simulink model "projectCE1_v2"  (R2024a)
settings: Solver=VariableStepAuto  StartTime=0.0  StopTime=0.1  RelTol=1e-3
libraries: dspsrcs4 x9, dspfdesign x6, commanapbnd3 x3, commchan3 x1
settings Model: Creator=nagel  LastModifiedBy=nagel

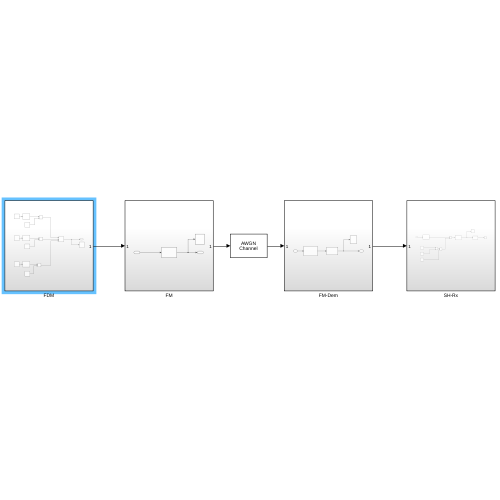
[thumbnail: Simulink's stored preview of the top-level diagram]
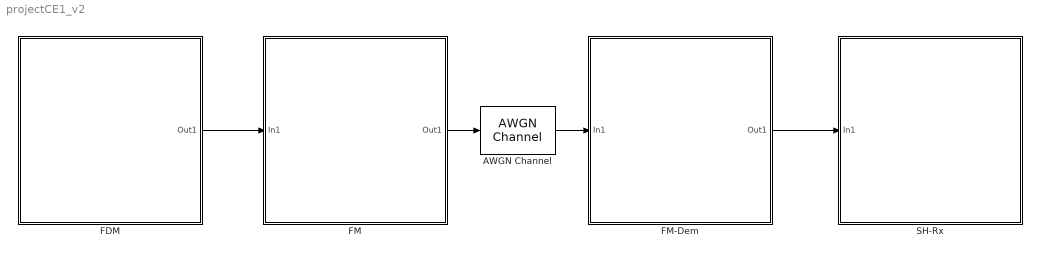
== system projectCE1_v2 ==
  AWGN Channel : commchan3/AWGN Channel  LegacyMode=off  NoiseMethod="Signal to noise ratio  (SNR)"  noiseMode="Signal to noise ratio  (SNR)"  EbNo=10  EsNo=10  SNR=10  BitsPerSymbol=1  SignalPower=1  SamplesPerSymbol=1  SymbolPeriod=1  VarianceSource=Parameter  Variance=1  RandomStream=mt19937ar with seed  Seed=67  SimulateUsing=Code generation
  FDM : Subsystem
  FM : Subsystem
  FM-Dem : Subsystem
  SH-Rx : Subsystem
  wires:
  FDM/1(Out1) -> FM/1(In1)
  FM/1(Out1) -> AWGN Channel/1
  AWGN Channel/1 -> FM-Dem/1(In1)
  FM-Dem/1(Out1) -> SH-Rx/1(In1)

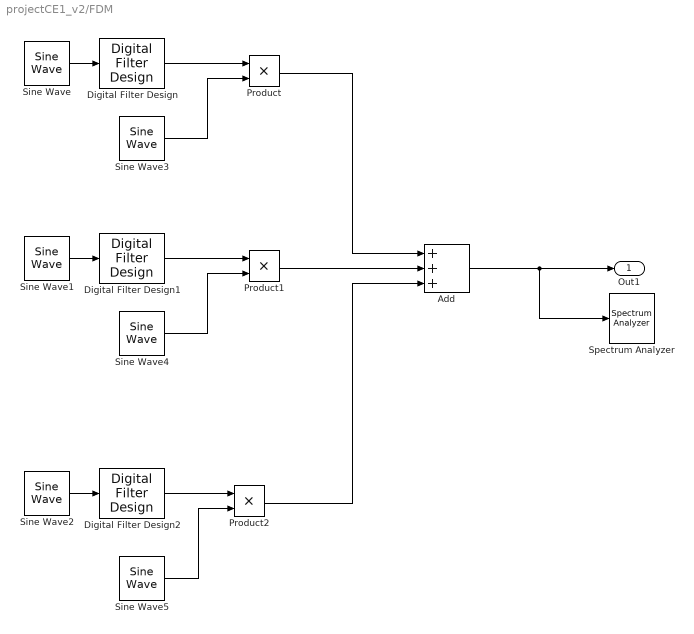
== system projectCE1_v2/FDM ==
  Add : Sum  Inputs=+++
  Digital Filter Design : dspfdesign/Digital Filter Design  mwdsp_browser_bugfix_var=off
  Digital Filter Design1 : dspfdesign/Digital Filter Design  mwdsp_browser_bugfix_var=off
  Digital Filter Design2 : dspfdesign/Digital Filter Design  mwdsp_browser_bugfix_var=off
  Product : Product
  Product1 : Product
  Product2 : Product
  Sine Wave : dspsrcs4/Sine Wave  Amplitude=1  Frequency=780  Phase=0  SampleMode=Discrete  OutComplex=Real  CompMethod=Trigonometric fcn  TableSize=Speed  SampleTime=1/(2*114e6)  SamplesPerFrame=1  ResetState=Restart at time zero  OutputFrames=off  dataType=double  wordLen=16  udDataType=sfix(16)  fracBitsMode=Best precision  numFracBits=15  OutDataTypeStr=double  LastOutDataTypeStr=double
  Sine Wave1 : dspsrcs4/Sine Wave  Amplitude=1  Frequency=4500  Phase=0  SampleMode=Discrete  OutComplex=Real  CompMethod=Trigonometric fcn  TableSize=Speed  SampleTime=1/(2*114e6)  SamplesPerFrame=1  ResetState=Restart at time zero  OutputFrames=off  dataType=double  wordLen=16  udDataType=sfix(16)  fracBitsMode=Best precision  numFracBits=15  OutDataTypeStr=double  LastOutDataTypeStr=double
  Sine Wave2 : dspsrcs4/Sine Wave  Amplitude=1  Frequency=10e3  Phase=0  SampleMode=Discrete  OutComplex=Real  CompMethod=Trigonometric fcn  TableSize=Speed  SampleTime=1/(2*114e6)  SamplesPerFrame=1  ResetState=Restart at time zero  OutputFrames=off  dataType=double  wordLen=16  udDataType=sfix(16)  fracBitsMode=Best precision  numFracBits=15  OutDataTypeStr=double  LastOutDataTypeStr=double
  Sine Wave3 : dspsrcs4/Sine Wave  Amplitude=1  Frequency=20e3  Phase=0  SampleMode=Discrete  OutComplex=Real  CompMethod=Trigonometric fcn  TableSize=Speed  SampleTime=1/(2*114e6)  SamplesPerFrame=1  ResetState=Restart at time zero  OutputFrames=off  dataType=double  wordLen=16  udDataType=sfix(16)  fracBitsMode=Best precision  numFracBits=15  OutDataTypeStr=double  LastOutDataTypeStr=double
  Sine Wave4 : dspsrcs4/Sine Wave  Amplitude=1  Frequency=60e3  Phase=0  SampleMode=Discrete  OutComplex=Real  CompMethod=Trigonometric fcn  TableSize=Speed  SampleTime=1/(2*114e6)  SamplesPerFrame=1  ResetState=Restart at time zero  OutputFrames=off  dataType=double  wordLen=16  udDataType=sfix(16)  fracBitsMode=Best precision  numFracBits=15  OutDataTypeStr=double  LastOutDataTypeStr=double
  Sine Wave5 : dspsrcs4/Sine Wave  Amplitude=1  Frequency=100e3  Phase=0  SampleMode=Discrete  OutComplex=Real  CompMethod=Trigonometric fcn  TableSize=Speed  SampleTime=1/(2*114e6)  SamplesPerFrame=1  ResetState=Restart at time zero  OutputFrames=off  dataType=double  wordLen=16  udDataType=sfix(16)  fracBitsMode=Best precision  numFracBits=15  OutDataTypeStr=double  LastOutDataTypeStr=double
  Spectrum Analyzer : SpectrumAnalyzer  WindowPosition=[372.000000,110.000000,1132.000000,588.000000,]  ScopeFrameLocation=window  SampleRate=44.1e3  PlotAsTwoSidedSpectrum=off  FrequencyScale=Log  FrequencySpan=Start and stop frequencies  Span=250e3  CenterFrequency=125e3  StartFrequency=0  StopFrequency=250e3  YLimits=[-44.5224692,27.38603855]
  Out1 : Outport
  wires:
  Sine Wave1/1 -> Digital Filter Design1/1
  Add/1 -> Out1/1, Spectrum Analyzer/1
  Sine Wave2/1 -> Digital Filter Design2/1
  Sine Wave/1 -> Digital Filter Design/1
  Digital Filter Design/1 -> Product/1
  Sine Wave3/1 -> Product/2
  Product/1 -> Add/1
  Digital Filter Design1/1 -> Product1/1
  Sine Wave4/1 -> Product1/2
  Product1/1 -> Add/2
  Sine Wave5/1 -> Product2/2
  Digital Filter Design2/1 -> Product2/1
  Product2/1 -> Add/3

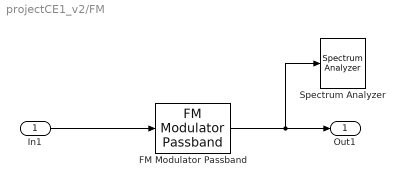
== system projectCE1_v2/FM ==
  In1 : Inport
  FM Modulator Passband : commanapbnd3/FM Modulator Passband  Fc=110e6  Ph=0  Kc=72e3
  Spectrum Analyzer : SpectrumAnalyzer  WindowPosition=[160.000000,154.000000,800.000000,500.000000,]  ScopeFrameLocation=window  RBWSource=Property  RBW=1e3  Span=227999999.99999997  StartFrequency=-113999999.99999999  StopFrequency=113999999.99999999  YLimits=[-99.98487156,25.09852185]
  Out1 : Outport
  wires:
  FM Modulator Passband/1 -> Spectrum Analyzer/1, Out1/1
  In1/1 -> FM Modulator Passband/1

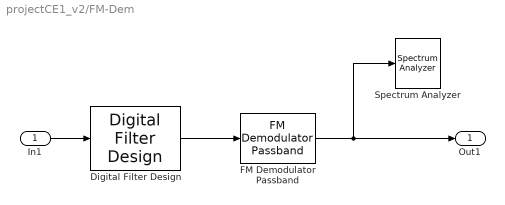
== system projectCE1_v2/FM-Dem ==
  In1 : Inport
  Digital Filter Design : dspfdesign/Digital Filter Design  mwdsp_browser_bugfix_var=off
  FM Demodulator Passband : commanapbnd3/FM Demodulator Passband  Fc=110e6  Ph=0  Kc=72e3  Ho=100
  Spectrum Analyzer : SpectrumAnalyzer  WindowPosition=[1027.000000,111.000000,800.000000,500.000000,]  ScopeFrameLocation=window  RBWSource=Property  RBW=1e3  Span=227999999.99999997  StartFrequency=-113999999.99999999  StopFrequency=113999999.99999999  YLimits=[-75.2783199,28.10619053]
  Out1 : Outport
  wires:
  In1/1 -> Digital Filter Design/1
  Digital Filter Design/1 -> FM Demodulator Passband/1
  FM Demodulator Passband/1 -> Spectrum Analyzer/1, Out1/1

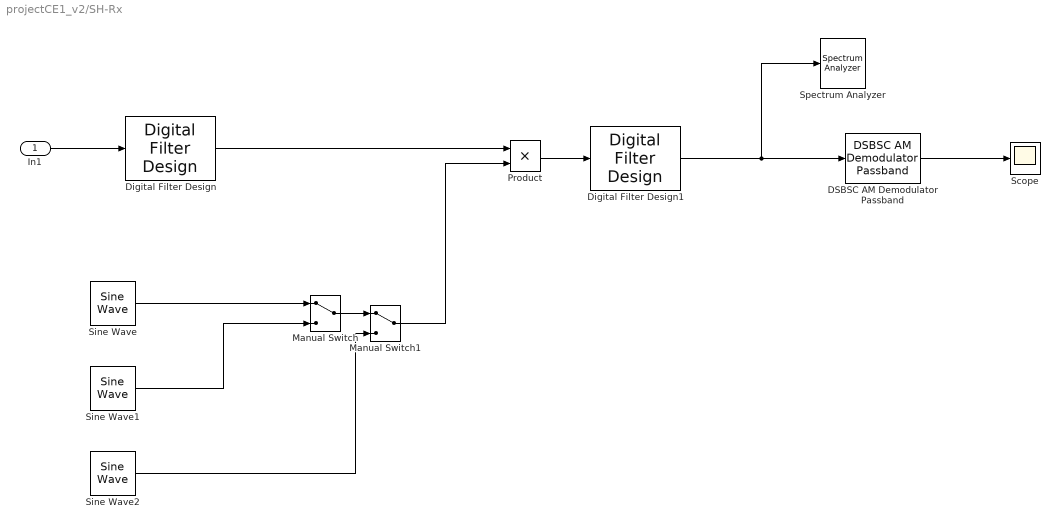
== system projectCE1_v2/SH-Rx ==
  In1 : Inport
  DSBSC AM Demodulator Passband : commanapbnd3/DSBSC AM Demodulator Passband  Fc=10.7e6  Ph=0  method=Butterworth  n=4  cf=15e3  Rp=0.1  Rs=50
  Digital Filter Design : dspfdesign/Digital Filter Design  mwdsp_browser_bugfix_var=off
  Digital Filter Design1 : dspfdesign/Digital Filter Design  mwdsp_browser_bugfix_var=off
  Manual Switch : ManualSwitch
  Manual Switch1 : ManualSwitch
  Product : Product
  Scope : Scope
  Sine Wave : dspsrcs4/Sine Wave  Amplitude=1  Frequency=10.7e6-20e3  Phase=0  SampleMode=Discrete  OutComplex=Real  CompMethod=Trigonometric fcn  TableSize=Speed  SampleTime=1/(2*114e6)  SamplesPerFrame=1  ResetState=Restart at time zero  OutputFrames=off  dataType=double  wordLen=16  udDataType=sfix(16)  fracBitsMode=Best precision  numFracBits=15  OutDataTypeStr=double  LastOutDataTypeStr=double
  Sine Wave1 : dspsrcs4/Sine Wave  Amplitude=1  Frequency=10.7e6-60e3  Phase=0  SampleMode=Discrete  OutComplex=Real  CompMethod=Trigonometric fcn  TableSize=Speed  SampleTime=1/(2*114e6)  SamplesPerFrame=1  ResetState=Restart at time zero  OutputFrames=off  dataType=double  wordLen=16  udDataType=sfix(16)  fracBitsMode=Best precision  numFracBits=15  OutDataTypeStr=double  LastOutDataTypeStr=double
  Sine Wave2 : dspsrcs4/Sine Wave  Amplitude=1  Frequency=10.7e6-100e3  Phase=0  SampleMode=Discrete  OutComplex=Real  CompMethod=Trigonometric fcn  TableSize=Speed  SampleTime=1/(2*114e6)  SamplesPerFrame=1  ResetState=Restart at time zero  OutputFrames=off  dataType=double  wordLen=16  udDataType=sfix(16)  fracBitsMode=Best precision  numFracBits=15  OutDataTypeStr=double  LastOutDataTypeStr=double
  Spectrum Analyzer : SpectrumAnalyzer  WindowPosition=[295.000000,189.000000,800.000000,500.000000,]  ScopeFrameLocation=window  RBWSource=Property  RBW=1e3  FrequencySpan=Start and stop frequencies  Span=30e3  CenterFrequency=10.7e6  StartFrequency=10.685e6  StopFrequency=10.715e6  YLimits=[-96.87272325,16.7371639]
  wires:
  Sine Wave/1 -> Manual Switch/1
  Sine Wave1/1 -> Manual Switch/2
  Manual Switch/1 -> Manual Switch1/1
  Sine Wave2/1 -> Manual Switch1/2
  Manual Switch1/1 -> Product/2
  Product/1 -> Digital Filter Design1/1
  Digital Filter Design1/1 -> DSBSC AM Demodulator Passband/1, Spectrum Analyzer/1
  DSBSC AM Demodulator Passband/1 -> Scope/1
  In1/1 -> Digital Filter Design/1
  Digital Filter Design/1 -> Product/1
